simulink model "EKF_unit_test"  (R2024a)
settings: Solver=VariableStepAuto  StartTime=0.0  StopTime=6  RelTol=1e-3
libraries: autolibshared x2, sim3dautolib x2, simulink_extras x2, sim3dprobsensorlib x2, trackingutilitieslib x1, dspstat3 x1, drivinglib x1, dspsigops x1, sim3dcameralib x1, sim3dphyssensorlib x1, sim3dlib x1, drivingsim3d x1
settings Model: Creator=moata  LastModifiedBy=moata

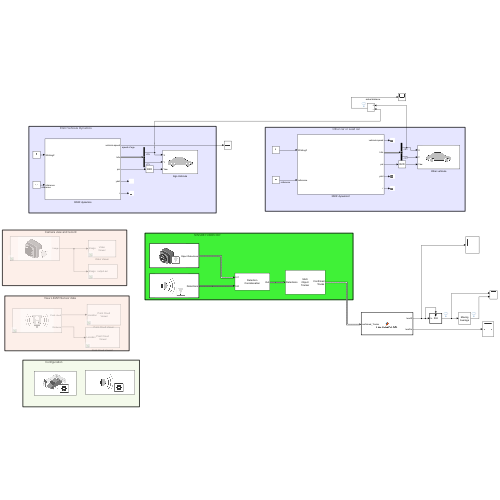
[thumbnail: Simulink's stored preview of the top-level diagram]
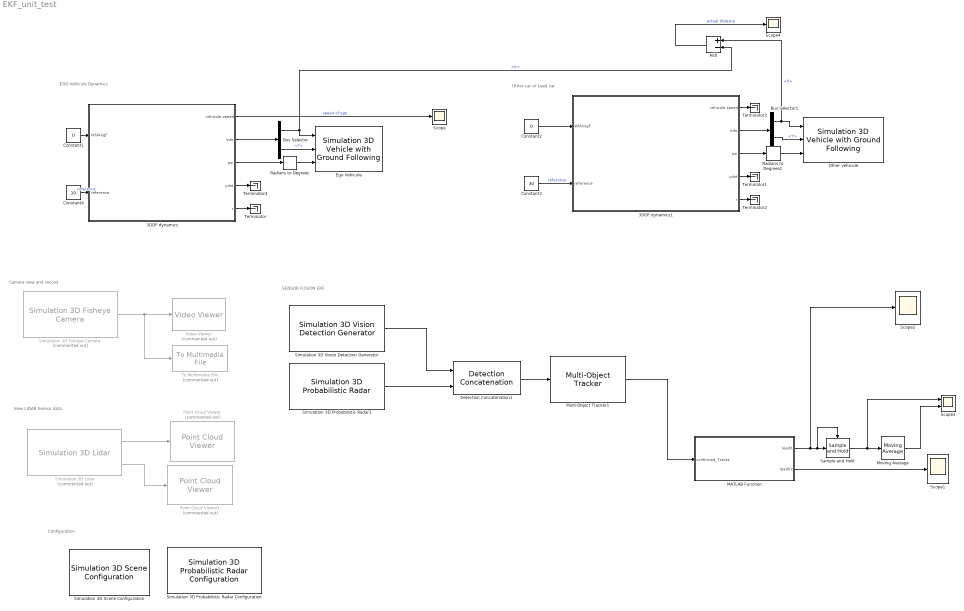
== system EKF_unit_test ==
  note: Other car or Lead car
  note: EGO Vehicule Dynamics
  note: Camera view and record
  note: View LIDAR Sensor data
  note: Configuration
  note: SENSOR FUSION EKF
  3DOF dynamics : Subsystem
  3DOF dynamics1 : Subsystem
  Add : Sum  Inputs=+-
  Bus Selector : BusSelector  OutputSignals=InertFrm.Cg.Disp.X,InertFrm.Cg.Disp.Y
  Bus Selector1 : BusSelector  OutputSignals=InertFrm.Cg.Disp.X,InertFrm.Cg.Disp.Y
  Constant1 : Constant  Value=0
  Constant2 : Constant  Value=0
  Constant3 : Constant  Value=30
  Constant4 : Constant  Value=10
  Detection Concatenation1 : trackingutilitieslib/Detection Concatenation  NumInputs=2  BusNameSource=Auto  BusName=BusDetectionConcatenation  SimulateUsing=Interpreted execution
      settings: LibrarySourceBlock=drivinglib/Detection Concatenation
  Ego Vehicule : sim3dautolib/Simulation 3D Vehicle with Ground Following  Priority=-1  PassVehMesh=Muscle car  MeshPath=/MathWorksAutomotiveContent/Vehicles/Muscle/Meshes/SK_MuscleCar.SK_MuscleCar  TrackWidth=1.9  WheelBase=3  WheelRadius=0.35  VehColor=Red  InitialPos=[0, 0, 0]  InitialRot=[0, 0, 0]  ActorName=SimulinkVehicle1  SampleTime=-1  ActorType=SimulinkVehicle  ID=1  aMode=3  ActorTag=SimulinkVehicle1  CoordinateScheme=ISO  VehLightsControl=off  HeadlightColor=[ 1, 1, 1 ]  HighBeamIntensity=100000  LowBeamIntensity=60000  HighBeamConeAngle=70  LowBeamConeAngle=70  LeftHeadlightOrientation=[ 0, 0 ]  RightHeadlightOrientation=[ 0, 0 ]  BrakelightIntensity=500  ReverselightIntensity=500  SignallightIntensity=500  SignallightPeriod=1  SignalPulseWidth=50  TransformOutportEnabled=off
      settings: LibrarySourceBlock=drivingsim3d/Simulation 3D Vehicle with Ground Following
  MATLAB Function : MATLAB Function  TreatAsAtomicUnit=on
  Moving Average : dspstat3/Moving Average  Method=Sliding window  ForgettingFactorPort=off  SpecifyWindowLength=on  WindowLength=20  OverlapLength=19  AllowArbitraryInputLength=off  ForgettingFactor=0.8  SimulateUsing=Interpreted execution
  Multi-Object Tracker1 : drivinglib/Multi-Object Tracker  TrackerIndex=uint32( 0 )  FilterInitializationFcn=initcvekf  AssignmentThreshold=30  ConfirmationThreshold=[ 2, 3 ]  DeletionThreshold=[ 5, 5 ]  MaxNumTracks=20  MaxNumSensors=2  OOSMHandling=Neglect  StateParametersSimulink=struct  HasStateParametersInput=off  TimeInputSource=Auto  HasCostMatrixInput=off  HasDetectableTrackIDsInput=off  BusNameSource=Property  BusName=BusMultiObjectTracker1  TentativeTracksOutputPort=off  AllTracksOutputPort=off  SimulateUsing=Interpreted execution
  Other vehicule : sim3dautolib/Simulation 3D Vehicle with Ground Following  Priority=-1  PassVehMesh=Box truck  MeshPath=/MathWorksAutomotiveContent/Vehicles/Muscle/Meshes/SK_MuscleCar.SK_MuscleCar  TrackWidth=1.9  WheelBase=3  WheelRadius=0.35  VehColor=Red  InitialPos=[30, 0, 0]  InitialRot=[0, 0, 0]  ActorName=SimulinkVehicle2  SampleTime=-1  ActorType=SimulinkVehicle  ID=2  aMode=3  ActorTag=SimulinkVehicle2  CoordinateScheme=ISO  VehLightsControl=off  HeadlightColor=[ 1, 1, 1 ]  HighBeamIntensity=100000  LowBeamIntensity=60000  HighBeamConeAngle=70  LowBeamConeAngle=70  LeftHeadlightOrientation=[ 0, 0 ]  RightHeadlightOrientation=[ 0, 0 ]  BrakelightIntensity=500  ReverselightIntensity=500  SignallightIntensity=500  SignallightPeriod=1  SignalPulseWidth=50  TransformOutportEnabled=off
      settings: LibrarySourceBlock=drivingsim3d/Simulation 3D Vehicle with Ground Following
  Point Cloud Viewer : PointCloudViewer  Commented=on  FigPos=[989.8 733.2 409.6 300]
  Point Cloud Viewer1 : PointCloudViewer  Commented=on  FigPos=[989.8 733.2 409.6 300]
  Radians to Degrees : simulink_extras/Transformations/Radians to Degrees
  Radians to Degrees1 : simulink_extras/Transformations/Radians to Degrees
  Sample and Hold : dspsigops/Sample and Hold  trig=Rising edge  initCond=0  latchinput=off
  Scope{,1..2,4} (4 alike) : Scope
  Scope3 : Scope  NumInputPorts=2
  Simulation 3D Fisheye Camera : sim3dcameralib/Simulation 3D Fisheye Camera  Priority=1  Commented=on  sensorTag=Sim3dSensor10  sensorId=10  sensorName=Sim3dSensor10  vehTagList={'Scene Origin';'SimulinkVehicle1';'SimulinkVehicle2'}  vehTag=SimulinkVehicle1  mountLoc=Front bumper  offsetFlag=off  tmountOffset=[0, 0, 0]  extTmount=off  rmountOffset=[0, 0, 0]  extRmount=off  OpticalCenter=[640, 360]  ImageSize=[720, 1280]  RadialDistortion=[320, 0, 0, 0]  StretchMatrix=[1, 0; 0, 1]  TransformOutportEnabled=off  SampleTime=-1  mountPoint=[2.47350001335144 0 0.439999997615814]  mountOrientation=[0 0 0]  aMode=3  ID=10
      settings: LibrarySourceBlock=drivingsim3d/Simulation 3D Fisheye Camera
  Simulation 3D Lidar : sim3dphyssensorlib/Simulation 3D Lidar  Priority=1  Commented=on  sensorTag=Sim3dSensor11  sensorId=11  sensorName=Sim3dSensor11  vehTagList={'Scene Origin';'SimulinkVehicle1';'SimulinkVehicle2'}  vehTag=SimulinkVehicle1  mountLoc=Hood center  offsetFlag=off  tmountOffset=[0, 0, 0]  rmountOffset=[0, 0, 0]  DetectionRange=120  RangeResolution=0.002  VerticalFOV=40  VerticalResolution=1.25  HorizontalFOV=360  HorizontalResolution=0.16  DistanceOutportEnabled=on  ReflectivityOutportEnabled=off  SemanticOutportEnabled=off  TransformOutportEnabled=off  SampleTime=-1  mountPoint=[1.27600002288818 0 1.12999999523163]  mountOrientation=[0 0 0]  aMode=3  ID=11
      settings: LibrarySourceBlock=drivingsim3d/Simulation 3D Lidar
  Simulation 3D Probabilistic Radar Configuration : sim3dprobsensorlib/Simulation 3D Probabilistic Radar Configuration  RCSactorKeys=[10]  RCSactorProfiles={[20, 25 ; 15, 30]}  RCSdefaultValue=-20  aMode=3
      settings: LibrarySourceBlock=drivingsim3d/Simulation 3D Probabilistic Radar Configuration
  Simulation 3D Probabilistic Radar1 : sim3dprobsensorlib/Simulation 3D Probabilistic Radar  Priority=1  sensorTag=Sim3dSensor12  sensorId=12  sensorName=Sim3dSensor12  vehTagList={'Scene Origin';'SimulinkVehicle1';'SimulinkVehicle2'}  vehTag=SimulinkVehicle1  mountLoc=Front bumper  offsetFlag=off  tmountOffset=[0, 0, 0]  rmountOffset=[0, 0, 0]  AzimuthResolution=4  ElevationResolution=5  RangeResolution=2.5  RangeRateResolution=0.5  AzimuthBiasFraction=0.1  ElevationBiasFraction=0.1  RangeBiasFraction=0.05  RangeRateBiasFraction=0.05  FieldOfView=[ 20, 5 ]  DetectionRange=[ 1, 500 ]  RangeRateLimits=[ -100, 100 ]  DetectionProbability=0.95  FalseAlarmRate=1e-7  ReferenceRange=500  ReferenceRCS=20  HasElevation=on  HasRangeRate=on  HasNoise=off  HasFalseAlarms=off  InitialSeedSource=Repeatable  InitialSeed=0  MaxNumDetections=150  DetectionCoordinates=Ego Cartesian  SpecifyOutputBusName=off  BusName=BusSimulation3DRadarTruthSensor  SampleTime=-1  mountPoint=[2.47350001335144 0 0.439999997615814]  mountOrientation=[0 0 0]  aMode=3  ID=12
      settings: LibrarySourceBlock=drivingsim3d/Simulation 3D Probabilistic Radar
  Simulation 3D Scene Configuration : sim3dlib/Simulation 3D Scene Configuration  Priority=0  ProjectFormat=Default Scenes  SceneDesc=Straight road  ProjectName=C:\Program Files\MATLAB\R2024a\toolbox\shared\sim3d_projects\automotive_project_windows\UE\WindowsNoEditor\VehicleSimulation.exe  ScenePath=/Game/Maps/HwStrght  EnableOpenDRIVE=off  vehTagList={'Custom';'Scene Origin';'SimulinkVehicle1';'SimulinkVehicle2'}  vehTag=Scene Origin  FreeCameraInitialTranslation=[0, 0, 0]  FreeCameraDefaultInitialTranslation=[-6, 0, 2]  FreeCameraInitialRotation=[0, 0, 0]  FreeCameraDefaultInitialRotation=[0, -15, 0]  OpVisEn=off  Ts=1/60  EnableWindow=on  EnableRemoteAccess=off  EnableWeather=off  SunAzimuth=90  SunAltitude=40.0  EnableGeospatialSun=off  Latitude=0  Longitude=0  Date=2023-01-01  Time=10:30:00  GeoTimeZone=-5.0  SunDaylightSaving=off  wind=1  clouds=10  EnableVolumetricClouds=off  CloudCoverage=0  CloudAltitude=6  fog=0  rain=0  RaindropsEffect=off  SnowDensity=0  EnableGeospatial=off  UseTrueOrigin=off  OriginHeight=200  OriginLatitude=40.744652  OriginLongitude=-73.988864  MapStyle=Aerial  AdditionalAssetIDs=[]  UseAdvancedSunSky=off  SolarTime=11  TimeZone=-5  Day=21  Month=9  Year=2022  UseDaylightSavingTime=on  DSTStartDay=10  DSTStartMonth=3  DSTEndDay=3  DSTEndMonth=11  DSTSwitchHour=2  sensorTag=MainCamera1  sensorId=1  sensorName=MainCamera1  mountLoc=Origin  offsetFlag=off  tmountOffset=[0, 0, 0]  rmountOffset=[0, 0, 0]  HorizontalResolution=1280  VerticalResolution=720  HorizontalFOV=60  mountPoint=[0 0 0]  mountOrientation=[0 0 0]  aMode=3  ID=1  GeoTrigger=Inactive
      settings: LibrarySourceBlock=drivingsim3d/Simulation 3D Scene Configuration
  Simulation 3D Vision Detection Generator : drivingsim3d/Simulation 3D Vision Detection Generator  Priority=1  sensorTag=Sim3dSensor255  sensorId=2  sensorName=Sim3dSensor2  vehTagList={'Scene Origin';'SimulinkVehicle1';'SimulinkVehicle2'}  vehTag=SimulinkVehicle1  mountLoc=Front bumper  offsetFlag=off  tmountOffset=[0, 0, 0]  rmountOffset=[0, 0, 0]  DetectorOutput=Objects only  MaxNumDetections=50  MaxNumLanes=30  laneSampleDistances=0:0.5:9.5  BusNameSource=Auto  BusName=BusObjectDetections  BusName2Source=Auto  BusName2=BusLaneDetections  MaxRange=500  BoundingBoxAccuracy=5  ProcessNoiseIntensity=5  MaxSpeed=50  MaxAllowedOcclusion=0.5  MinObjectImageSize=[ 15, 15 ]  DetectionProbability=0.9  FalsePositivesPerImage=0  MinLaneImageSize=[ 20, 3 ]  LaneBoundaryAccuracy=3  HasNoise=off  InitialSeedSource=Repeatable  InitialSeed=1  uniqueActorIdentifier=[]  actorClassInteger=0  cuboidLength=4.7  cuboidWidth=1.8  cuboidHeight=1.4  rotationalCenter={[-1.35, 0, 0]}  focalLength=[800, 800]  opticalCenter=[320, 240]  imageSize=[480, 640]  radialDistortionCoefficients=[0, 0]  tangentialDistortionCoefficients=[0, 0]  cameraAxisSkew=0  actorTruthOutportEnabled=off  laneTruthOutportEnabled=off  SampleTime=-1  checkedSampleTime=0.016667  mountPoint=[2.47350001335144 0 0.439999997615814]  mountOrientation=[0 0 0]  aMode=3  ID=2
  Terminator{,1..4} (5 alike) : Terminator
  To Multimedia File : dspvision/To Multimedia File  Commented=on  outputFilename=C:\Users\moata\Desktop\output.avi  streamSelection=Video only  videoCompressor=None (uncompressed)  audioCompressor=None (uncompressed)  imagePorts=One multidimensional signal  fileType=AVI  audioDatatype=Determine from input data type  fourcc=RGB  audioBitRate=128  audioQuality=75  videoQuality=75  mj2000CompFactor=10
      settings: LibrarySourceBlock=visionsinks/To Multimedia File
  Video Viewer : VideoViewer  Commented=on  FigPos=[931.4 762.8 482.4 364.8]
  wires:
  Bus Selector/1 -> Add/2, Ego Vehicule/1  "<X>"
  Bus Selector/2 -> Ego Vehicule/2  "<Y>"
  Simulation 3D Fisheye Camera/1 -> Video Viewer/1, To Multimedia File/1
  Simulation 3D Lidar/1 -> Point Cloud Viewer/1
  Constant1/1 -> 3DOF dynamics/1(WhlAngF)
  3DOF dynamics/2(Info) -> Bus Selector/1
  3DOF dynamics/3(psi) -> Radians to Degrees/1
  3DOF dynamics/4(ydot) -> Terminator4/1
  3DOF dynamics/5(r) -> Terminator/1
  Simulation 3D Lidar/2 -> Point Cloud Viewer1/1
  3DOF dynamics1/2(Info) -> Bus Selector1/1
  Bus Selector1/1 -> Add/1, Other vehicule/1  "<X>"
  Bus Selector1/2 -> Other vehicule/2  "<Y>"
  3DOF dynamics1/3(psi) -> Radians to Degrees1/1
  3DOF dynamics1/4(ydot) -> Terminator1/1
  3DOF dynamics1/5(r) -> Terminator2/1
  3DOF dynamics1/1(vehicule speed) -> Terminator3/1
  Constant2/1 -> 3DOF dynamics1/1(WhlAngF)
  Constant3/1 -> 3DOF dynamics1/2(reference)  "reference"
  3DOF dynamics/1(vehicule speed) -> Scope/1  "speed of ego"
  Constant4/1 -> 3DOF dynamics/2(reference)  "reference"
  Radians to Degrees/1 -> Ego Vehicule/3
  Radians to Degrees1/1 -> Other vehicule/3
  Multi-Object Tracker1/1 -> MATLAB Function/1(confirmed_Tracks)
  MATLAB Function/2(leadVx) -> Scope1/1
  MATLAB Function/1(leadX) -> Sample and Hold/Trigger, Sample and Hold/1, Scope2/1
  Sample and Hold/1 -> Scope3/1, Moving Average/1
  Moving Average/1 -> Scope3/2
  Add/1 -> Scope4/1  "actual distance"
  Simulation 3D Vision Detection Generator/1 -> Detection Concatenation1/1
  Detection Concatenation1/1 -> Multi-Object Tracker1/1
  Simulation 3D Probabilistic Radar1/1 -> Detection Concatenation1/2

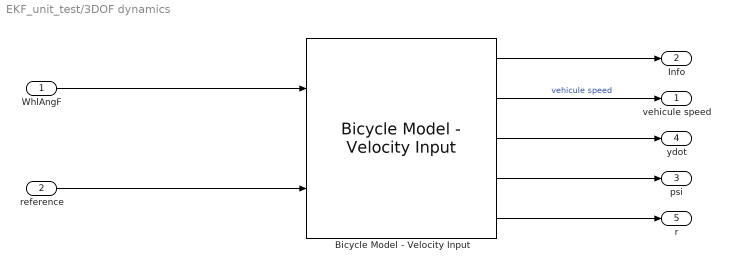
== system EKF_unit_test/3DOF dynamics ==
  WhlAngF : Inport
  reference : Inport  Port=2
  Bicycle Model - Velocity Input : autolibshared/Bicycle Model - Velocity Input  trackMode=Single (bicycle)  inputMode=External longitudinal velocity  frontSteerMode=on  rearSteerMode=off  windMode=off  muMode=off  extFMode=off  extMMode=off  aMode=3  NF=2  NR=2  m=2000  a=1.4  b=1.6  h=0.35  X_o=0  xdot_o=0  CalphaMode=off  sigmaMode=on  w=[1.4,1.4]  Cy_f=12e3  Cy_r=11e3  sigma_f=.1  sigma_r=.1  alpha_f_brk=[-.1 .1]  Cy_f_data=[-9e3 9e3]  alpha_r_brk=[-.1 .1]  Cy_r_data=[-9e3 9e3]  Y_o=0  ydot_o=0  Izz=4000  psi_o=0  r_o=0  Af=2  Cd=.3  Cl=.1  Cpm=.1  beta_w=[0 0.01:0.01:0.3]  Cs=[0 0.01:0.01:0.3]  Cym=[0 1e-6:0.01:0.3]  Pabs=101325  Tair=273  g=9.81  mu=1  xdot_tol=.01  Fznom=5000  Fxtire_sat=1e6  Fytire_sat=1e6  longOff=0  latOff=0  vertOff=0
      settings: LibrarySourceBlock=drivingscenarioandsensors/Bicycle Model - Velocity Input
  vehicule speed : Outport
  Info : Outport  Port=2
  psi : Outport  Port=3
  ydot : Outport  Port=4
  r : Outport  Port=5
  wires:
  Bicycle Model - Velocity Input/5 -> r/1
  Bicycle Model - Velocity Input/1 -> Info/1
  reference/1 -> Bicycle Model - Velocity Input/2
  Bicycle Model - Velocity Input/4 -> psi/1
  Bicycle Model - Velocity Input/3 -> ydot/1
  WhlAngF/1 -> Bicycle Model - Velocity Input/1
  Bicycle Model - Velocity Input/2 -> vehicule speed/1  "vehicule speed"

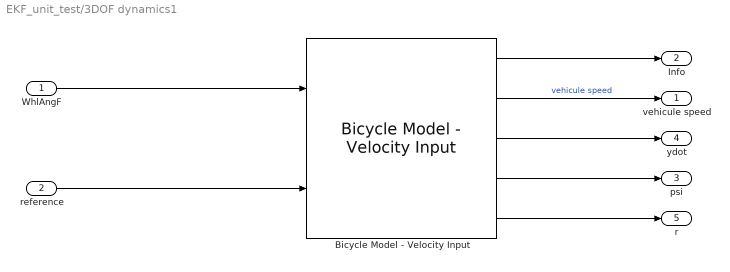
== system EKF_unit_test/3DOF dynamics1 ==
  WhlAngF : Inport
  reference : Inport  Port=2
  Bicycle Model - Velocity Input : autolibshared/Bicycle Model - Velocity Input  trackMode=Single (bicycle)  inputMode=External longitudinal velocity  frontSteerMode=on  rearSteerMode=off  windMode=off  muMode=off  extFMode=off  extMMode=off  aMode=3  NF=2  NR=2  m=2000  a=1.4  b=1.6  h=0.35  X_o=30  xdot_o=0  CalphaMode=off  sigmaMode=on  w=[1.4,1.4]  Cy_f=12e3  Cy_r=11e3  sigma_f=.1  sigma_r=.1  alpha_f_brk=[-.1 .1]  Cy_f_data=[-9e3 9e3]  alpha_r_brk=[-.1 .1]  Cy_r_data=[-9e3 9e3]  Y_o=0  ydot_o=0  Izz=4000  psi_o=0  r_o=0  Af=2  Cd=.3  Cl=.1  Cpm=.1  beta_w=[0 0.01:0.01:0.3]  Cs=[0 0.01:0.01:0.3]  Cym=[0 1e-6:0.01:0.3]  Pabs=101325  Tair=273  g=9.81  mu=1  xdot_tol=.01  Fznom=5000  Fxtire_sat=1e6  Fytire_sat=1e6  longOff=0  latOff=0  vertOff=0
      settings: LibrarySourceBlock=drivingscenarioandsensors/Bicycle Model - Velocity Input
  vehicule speed : Outport
  Info : Outport  Port=2
  psi : Outport  Port=3
  ydot : Outport  Port=4
  r : Outport  Port=5
  wires:
  Bicycle Model - Velocity Input/2 -> vehicule speed/1  "vehicule speed"
  WhlAngF/1 -> Bicycle Model - Velocity Input/1
  Bicycle Model - Velocity Input/3 -> ydot/1
  Bicycle Model - Velocity Input/4 -> psi/1
  reference/1 -> Bicycle Model - Velocity Input/2
  Bicycle Model - Velocity Input/1 -> Info/1
  Bicycle Model - Velocity Input/5 -> r/1

== matlab function EKF_unit_test/MATLAB Function ==
  data: confirmed_Tracks input; leadX output; leadVx output
function [leadX, leadVx] = extractLeadCarInfo(confirmed_Tracks)
    
    leadX = confirmed_Tracks.Tracks(1).State(1);
    leadVx = confirmed_Tracks.Tracks(1).State(2); % X velocity

end
